simulink model "Senales_B1"  (R2023a)
settings: Solver=VariableStepAuto  StartTime=0.0  StopTime=10  RelTol=1e-3
undefined symbols (not defined in the file or in its folder): DiscIntNeverNeededParam
settings Model: Creator=albsa  LastModifiedBy=albsa

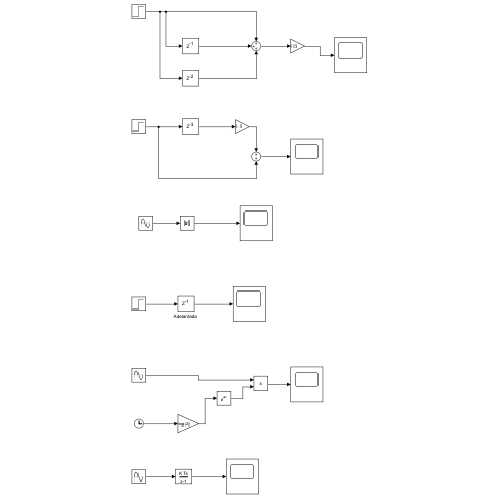
[thumbnail: Simulink's stored preview of the top-level diagram]
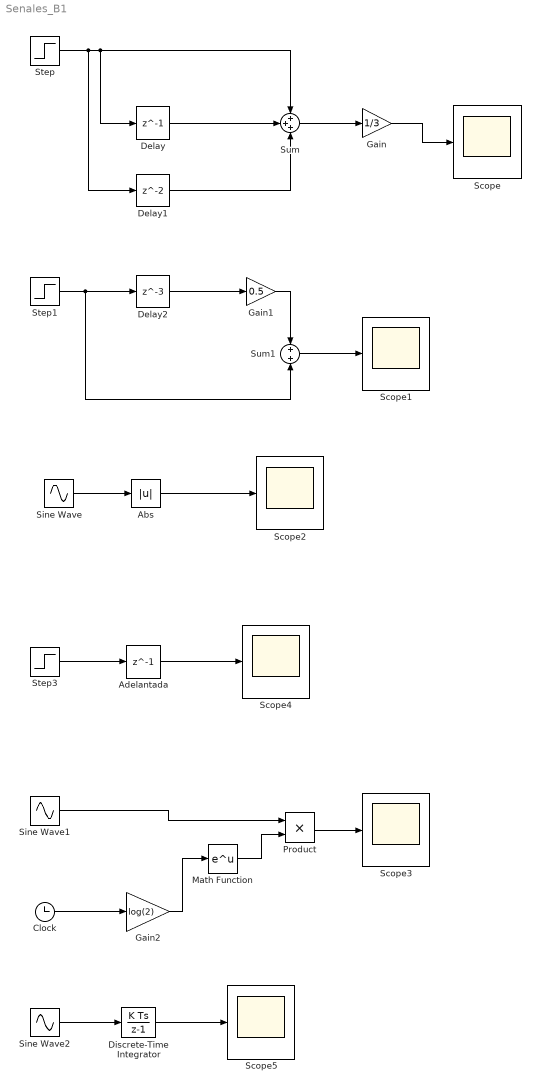
== system Senales_B1 ==
  Abs : Abs  SaturateOnIntegerOverflow=off
  "Adelantada " : Delay  DelayLength=1  InitialCondition=0  SampleTime=1
  Clock : Clock
  Delay : Delay  DelayLength=1  InitialCondition=0  SampleTime=1
  Delay1 : Delay  InitialCondition=0  SampleTime=1
  Delay2 : Delay  DelayLength=3  InitialCondition=0  SampleTime=1
  Discrete-Time Integrator : DiscreteIntegrator  SampleTime=-1  ICPrevOutput=DiscIntNeverNeededParam  ICPrevScaledInput=DiscIntNeverNeededParam
  Gain : Gain  Gain=1/3
  Gain1 : Gain  Gain=0.5
  Gain2 : Gain  Gain=log(2)
  Math Function : Math
  Product : Product
  Scope{,1..5} (6 alike) : Scope
  Sine Wave : Sin  Amplitude=2  SampleTime=0
  Sine Wave1 : Sin  Amplitude=2  SampleTime=0
  Sine Wave2 : Sin  Amplitude=2  SampleTime=0
  Step : Step  SampleTime=0
  Step1 : Step  SampleTime=0
  Step3 : Step  SampleTime=0
  Sum : Sum  Inputs=+++
  Sum1 : Sum
  wires:
  Step/1 -> Sum/1, Delay/1, Delay1/1
  Delay/1 -> Sum/2
  Delay1/1 -> Sum/3
  Sum/1 -> Gain/1
  Gain/1 -> Scope/1
  Step1/1 -> Sum1/2, Delay2/1
  Delay2/1 -> Gain1/1
  Gain1/1 -> Sum1/1
  Sum1/1 -> Scope1/1
  Sine Wave/1 -> Abs/1
  Abs/1 -> Scope2/1
  Step3/1 -> "Adelantada "/1
  "Adelantada "/1 -> Scope4/1
  Clock/1 -> Gain2/1
  Gain2/1 -> Math Function/1
  Math Function/1 -> Product/2
  Sine Wave1/1 -> Product/1
  Product/1 -> Scope3/1
  Sine Wave2/1 -> Discrete-Time Integrator/1
  Discrete-Time Integrator/1 -> Scope5/1
